simulink model "hw6_nonlinear_pendulum"  (R2026a)
settings: Solver=ode4  StopTime=5  FixedStep=0.005
model workspace (MAT data in the model file):
  I = 0.006
  M = 0.5
  b = 0.1
  g = 9.81
  l = 0.3
  m = 0.2
libraries: slpidlib x1
settings Model: Creator=ievge  LastModifiedBy=ievge

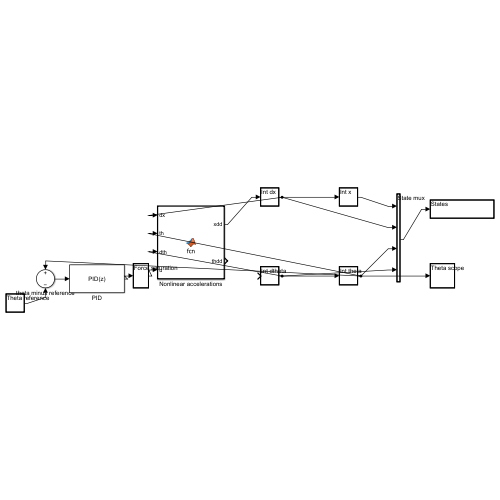
[thumbnail: Simulink's stored preview of the top-level diagram]
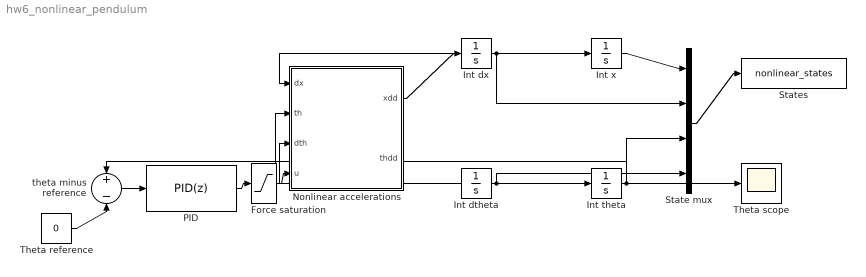
== system hw6_nonlinear_pendulum ==
  Force saturation : Saturate  UpperLimit=20  LowerLimit=-20
  Int dtheta : Integrator
  Int dx : Integrator
  Int theta : Integrator  InitialCondition=10*pi/180
  Int x : Integrator
  Nonlinear accelerations : MATLAB Function  TreatAsAtomicUnit=on
  PID : slpidlib/PID Controller  Controller=PID  Form=Parallel  TimeDomain=Discrete-time  UseExternalTs=off  SampleTime=0.005  IntegratorMethod=Forward Euler  FilterMethod=Forward Euler  ControllerParametersSource=internal  P=40  I=50  UseKiTs=off  D=5  UseExternalDerivativeSource=off  N=100  UseFilter=on  TunerSelectOption=Transfer Function Based (PID Tuner App)  InitialConditionSource=internal  InitialConditionForIntegrator=0  InitialConditionForFilter=0  DifferentiatorICPrevScaledInput=0  ExternalReset=none  TrackingMode=off  Kt=1  LimitOutput=off  SatLimitsSource=internal  UpperSaturationLimit=inf  LowerSaturationLimit=-inf  LinearizeAsGain=off  AntiWindupMode=none  Kb=1  LimitIntegrator=off  UpperIntegratorSaturationLimit=inf  LowerIntegratorSaturationLimit=-inf  POutMin=[]  POutMax=[]  IOutMin=[]  IOutMax=[]  DOutMin=[]  DOutMax=[]  NOutMin=[]  NOutMax=[]  SumOutMin=[]  SumOutMax=[]  SaturationOutMin=[]  SaturationOutMax=[]  PParamMin=[]  PParamMax=[]  IParamMin=[]  IParamMax=[]  DParamMin=[]  DParamMax=[]  NParamMin=[]  NParamMax=[]  KbParamMin=[]  KbParamMax=[]  KtParamMin=[]  KtParamMax=[]  KbOutMin=[]  KbOutMax=[]  KtOutMin=[]  KtOutMax=[]  IntegratorOutMin=[]  IntegratorOutMax=[]  FilterOutMin=[]  FilterOutMax=[]  SumI1OutMin=[]  SumI1OutMax=[]  SumI2OutMin=[]  SumI2OutMax=[]  SumI3OutMin=[]  SumI3OutMax=[]  SumI4OutMin=[]  SumI4OutMax=[]  SumDOutMin=[]  SumDOutMax=[]  DifferentiatorOutMin=[]  DifferentiatorOutMax=[]  FilterDiffOutCoefMin=[]  FilterDiffOutCoefMax=[]  ReciprocalOutMin=[]  ReciprocalOutMax=[]  SumDenOutMin=[]  SumDenOutMax=[]  SumNumOutMin=[]  SumNumOutMax=[]  DivideOutMin=[]  DivideOutMax=[]  UdiffTsProdOutMin=[]  UdiffTsProdOutMax=[]  NTsProdOutMin=[]  NTsProdOutMax=[]  UintegralTsProdOutMin=[]  UintegralTsProdOutMax=[]  UngainTsProdOutMin=[]  UngainTsProdOutMax=[]  ClampingZeroOutDataTypeStr=Inherit: Inherit via back propagation  ClampingZeroOutMin=[]  ClampingZeroOutMax=[]  FilterDenConstantOutDataTypeStr=Inherit: Inherit via back propagation  FilterDenConstantOutMin=[]  FilterDenConstantOutMax=[]  PCopyOutDataTypeStr=Inherit: Inherit via back propagation  PCopyOutMin=[]  PCopyOutMax=[]  NCopyOutDataTypeStr=Inherit: Inherit via back propagation  NCopyOutMin=[]  NCopyOutMax=[]  IntegratorContinuousStateAttributes=''  IntegratorStateMustResolveToSignalObject=off  IntegratorRTWStateStorageClass=Auto  FilterContinuousStateAttributes=''  FilterStateMustResolveToSignalObject=off  FilterRTWStateStorageClass=Auto  ParallelPVariant=InternalParameters  IdealPVariant=Disabled  IVariant=InternalParameters  DVariant=InternalParameters  IntegratorVariant=Discrete  SatVariant=Disabled  AWVariant=Passthrough  PCopyVariant=Disabled  TRVariant=Disabled  FdbkBlocksVariant=Forward  IdealPFdbkVariant=Disabled  SatFdbkVariant=Disabled  DerivativeFilterVariant=ForwardEulerFilter  NVariant=InternalParameters  NCopyVariant=Disabled  FilterICVariant=InternalICsFilter  IntegratorICVariant=InternalICs  ExternalResetVariant=Disabled  TRSumVariant=Passthrough  SumFdbkVariant=Disabled  SumVariant=Sum_PID  TsampFilterVariant=InternalTs  TsampNgainVariant=Passthrough  TsampIntegralVariant=Disabled_SignalSpec  ExternalSaturationOutDataTypeStr=Inherit: Same as second input  DerivativeSourceVariant=ErrorSignal  PreIntVariant=InternalPreInt
      settings: LibrarySourceBlock=simulink/Discrete/Discrete PID Controller
  State mux : Mux
  States : ToWorkspace  VariableName=nonlinear_states  SaveFormat=Structure With Time  SampleTime=-1
  Theta reference : Constant  Value=0
  Theta scope : Scope
  theta minus reference : Sum  Inputs=+-
  wires:
  Int dx/1 -> Int x/1, Nonlinear accelerations/1(dx), State mux/2
  Int x/1 -> State mux/1
  Nonlinear accelerations/1(xdd) -> Int dx/1
  Int dtheta/1 -> Int theta/1, Nonlinear accelerations/3(dth), State mux/4
  Int theta/1 -> theta minus reference/1, Nonlinear accelerations/2(th), State mux/3, Theta scope/1
  Theta reference/1 -> theta minus reference/2
  theta minus reference/1 -> PID/1
  PID/1 -> Force saturation/1
  Force saturation/1 -> Nonlinear accelerations/4(u)
  State mux/1 -> States/1

== matlab function hw6_nonlinear_pendulum/Nonlinear accelerations ==
  data: dx input; th input; dth input; u input; xdd output; thdd output
function [xdd,thdd] = fcn(dx,th,dth,u)
%#codegen
M = 0.5; m = 0.2; b = 0.1; l = 0.3; I = 0.006; g = 9.81;
c = cos(th); s = sin(th);
detA = (M+m)*(I+m*l^2) - (m*l*c)^2;
rhs1 = u - b*dx + m*l*dth^2*s; rhs2 = m*g*l*s;
xdd = ((I+m*l^2)*rhs1 - m*l*c*rhs2)/detA;
thdd = (-(m*l*c)*rhs1 + (M+m)*rhs2)/detA;
end
